simulink model "MATLAB_Function"  (R2025b)
settings: Solver=VariableStepAuto  StartTime=0.0  StopTime=10.0  MaxStep=0.01  RelTol=1e-3
settings Model: Creator=night  LastModifiedBy=night

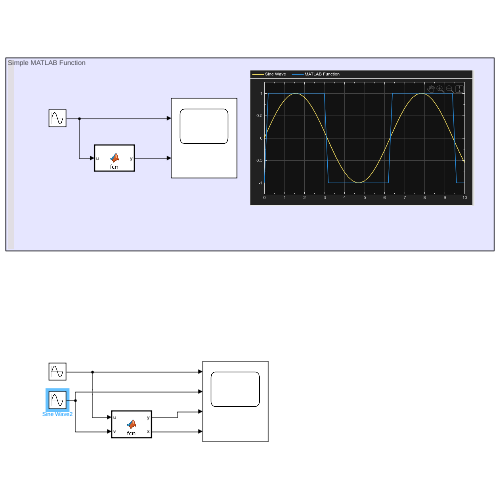
[thumbnail: Simulink's stored preview of the top-level diagram]
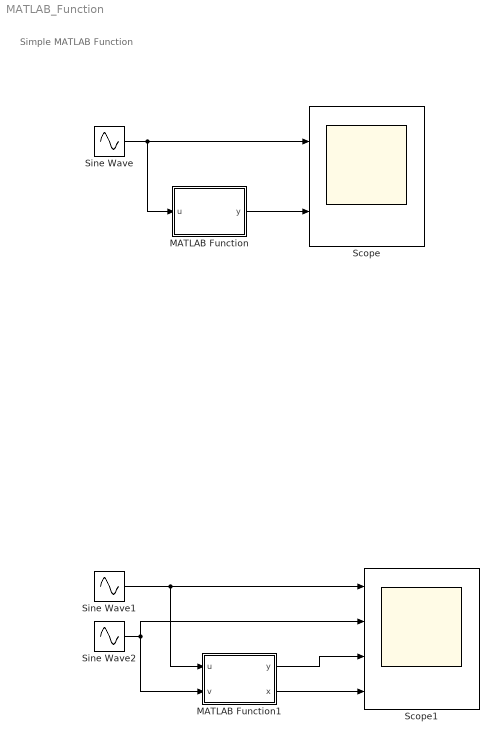
== system MATLAB_Function ==
  note: Simple MATLAB Function
  MATLAB Function : MATLAB Function  TreatAsAtomicUnit=on
  MATLAB Function1 : MATLAB Function  TreatAsAtomicUnit=on
  Scope : Scope  NumInputPorts=2
      settings: ActiveDisplayYMinimum=-1.2456318853205086  ActiveDisplayYMaximum=1.2490408795261734
  Scope1 : Scope  NumInputPorts=4
      settings: ActiveDisplayYMinimum=-1.7677258255930697  ActiveDisplayYMaximum=1.7677423790464708
  Sine Wave : Sin  Frequency=2  SampleTime=0
  Sine Wave1 : Sin  Frequency=2  SampleTime=0
  Sine Wave2 : Sin  Frequency=2  Phase=pi/2  SampleTime=0
  wires:
  Sine Wave/1 -> MATLAB Function/1(u), Scope/1
  MATLAB Function/1(y) -> Scope/2
  Sine Wave1/1 -> MATLAB Function1/1(u), Scope1/1
  Sine Wave2/1 -> Scope1/2, MATLAB Function1/2(v)
  MATLAB Function1/1(y) -> Scope1/3
  MATLAB Function1/2(x) -> Scope1/4

== matlab function MATLAB_Function/MATLAB Function ==
  data: u input; y output
function y = fcn(u)
if u > 0
    y = 1;
else 
    y = -1
end

== matlab function MATLAB_Function/MATLAB Function1 ==
  data: u input; y output; v input; x output
function [y,x] = fcn(u,v)
if u > v
    y = 1;
    x = u + v;
else 
    y = 0;
    x = 0;
end
